simulink model "EScooter_Logical_Architecture"  (R2025b)
settings: Solver=VariableStepAuto  StartTime=0.0  StopTime=10.0  RelTol=1e-3
settings Model: Creator=louis  LastModifiedBy=louis

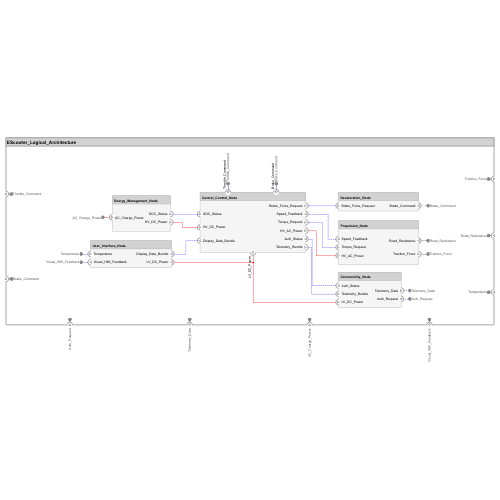
[thumbnail: Simulink's stored preview of the top-level diagram]
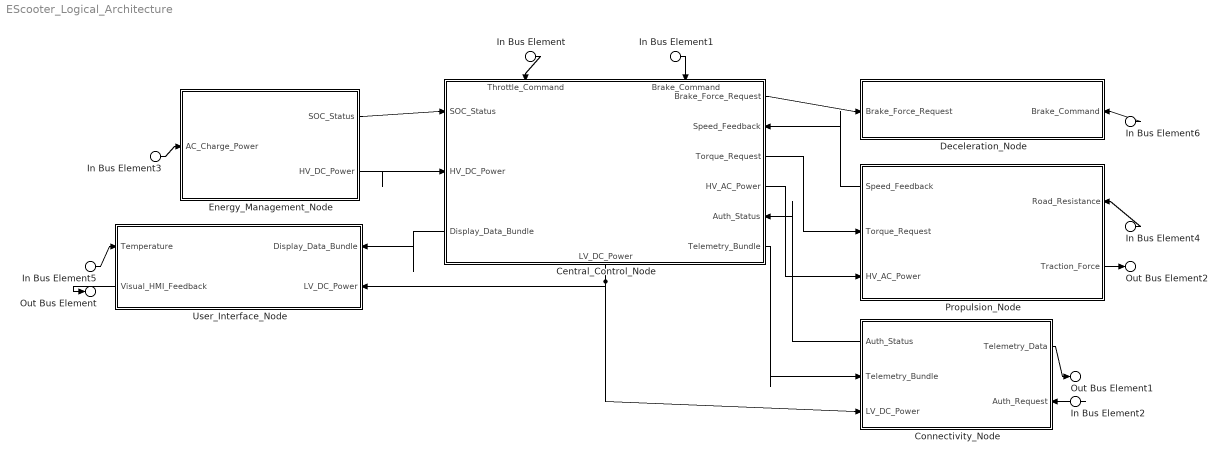
== system EScooter_Logical_Architecture ==
  In Bus Element : Inport  PortName=Throttle_Command
  In Bus Element6 : Inport  Port=2  PortName=Brake_Command
  In Bus Element1 : Inport  Port=2  PortName=Brake_Command
  In Bus Element2 : Inport  Port=3  PortName=Auth_Request
  In Bus Element3 : Inport  Port=4  PortName=AC_Charge_Power
  In Bus Element4 : Inport  Port=5  PortName=Road_Resistance
  In Bus Element5 : Inport  Port=6  PortName=Temperature
  Central_Control_Node : Subsystem
      settings: PortSchema="{\"entries\":[{\"content\":{\"headerSize\":26,\"margin\":15,\"minimumSpacing\":25,\"sides\":[{\"content\":{\"connectorIds\":[\"In6\",\"In3\",\"Out3\"]},\"type\":\"ConnectorPlacement.EquallySpacedRectSide\",\"uuid\":\"144652b9-dd85-470f-8014-e792da2fa2ac\"},{\"content\":{\"connectorIds\":[\"Out4\",\"In5\",\"Out6\",\"Out2\",\"In4\",\"Out5\"],\"side\":\"RIGHT\"},\"type\":\"ConnectorPlacement.EquallySpacedRectSide\",\"uuid\":\"d391e3f2-978f-4ccc-ab2b-52567d421a28\"},{\"content\":{\"connectorIds\":[\"In1\",\"In2\"],\"side\":\"TOP\"},\"type\":\"ConnectorPlacement.EquallySpacedRectSide\",\"uuid\":\"a45f99b3-1281-4051-bb9b-2205db18ec2a\"},{\"content\":{\"connectorIds\":[\"Out1\"],\"side\":\"BOTTOM\"},\"type\":\"ConnectorPlacement.EquallySpacedRectSide\",\"uuid\":\"be097ea3-5c6b-435f-9d5e-6a4f101ead8d\"}]},\"type\":\"ConnectorPlacement.EquallySpacedConnector\",\"uuid\":\"69c8647b-5d40-4da9-a90b-a75e053ae147\"}],\"packageUris\":[\"http://schema.mathworks.com/mf0/Connector/R2020b\"],\"version\":\"1.0\"}"
  Connectivity_Node : Subsystem
      settings: PortSchema="{\"entries\":[{\"content\":{\"headerSize\":26,\"margin\":15,\"minimumSpacing\":25,\"sides\":[{\"content\":{\"connectorIds\":[\"Out2\",\"In3\",\"In2\"]},\"type\":\"ConnectorPlacement.EquallySpacedRectSide\",\"uuid\":\"144652b9-dd85-470f-8014-e792da2fa2ac\"},{\"content\":{\"connectorIds\":[\"Out1\",\"In1\"],\"side\":\"RIGHT\"},\"type\":\"ConnectorPlacement.EquallySpacedRectSide\",\"uuid\":\"d391e3f2-978f-4ccc-ab2b-52567d421a28\"},{\"content\":{\"side\":\"TOP\"},\"type\":\"ConnectorPlacement.EquallySpacedRectSide\",\"uuid\":\"a45f99b3-1281-4051-bb9b-2205db18ec2a\"},{\"content\":{\"side\":\"BOTTOM\"},\"type\":\"ConnectorPlacement.EquallySpacedRectSide\",\"uuid\":\"4c3afbfa-e7d8-4b27-9477-116bc0ba0eb7\"}]},\"type\":\"ConnectorPlacement.EquallySpacedConnector\",\"uuid\":\"69c8647b-5d40-4da9-a90b-a75e053ae147\"}],\"packageUris\":[\"http://schema.mathworks.com/mf0/Connector/R2020b\"],\"version\":\"1.0\"}"
  Deceleration_Node : Subsystem
      settings: PortSchema="{\"entries\":[{\"content\":{\"headerSize\":26,\"margin\":15,\"minimumSpacing\":25,\"sides\":[{\"content\":{\"connectorIds\":[\"In2\"]},\"type\":\"ConnectorPlacement.EquallySpacedRectSide\",\"uuid\":\"144652b9-dd85-470f-8014-e792da2fa2ac\"},{\"content\":{\"connectorIds\":[\"In1\"],\"side\":\"RIGHT\"},\"type\":\"ConnectorPlacement.EquallySpacedRectSide\",\"uuid\":\"d391e3f2-978f-4ccc-ab2b-52567d421a28\"},{\"content\":{\"side\":\"TOP\"},\"type\":\"ConnectorPlacement.EquallySpacedRectSide\",\"uuid\":\"a45f99b3-1281-4051-bb9b-2205db18ec2a\"}]},\"type\":\"ConnectorPlacement.EquallySpacedConnector\",\"uuid\":\"69c8647b-5d40-4da9-a90b-a75e053ae147\"}],\"packageUris\":[\"http://schema.mathworks.com/mf0/Connector/R2020b\"],\"version\":\"1.0\"}"
  Energy_Management_Node : Subsystem
      settings: PortSchema="{\"entries\":[{\"content\":{\"headerSize\":26,\"margin\":15,\"minimumSpacing\":25,\"sides\":[{\"content\":{\"connectorIds\":[\"In1\"]},\"type\":\"ConnectorPlacement.EquallySpacedRectSide\",\"uuid\":\"144652b9-dd85-470f-8014-e792da2fa2ac\"},{\"content\":{\"connectorIds\":[\"Out1\",\"Out2\"],\"side\":\"RIGHT\"},\"type\":\"ConnectorPlacement.EquallySpacedRectSide\",\"uuid\":\"d391e3f2-978f-4ccc-ab2b-52567d421a28\"},{\"content\":{\"side\":\"TOP\"},\"type\":\"ConnectorPlacement.EquallySpacedRectSide\",\"uuid\":\"a45f99b3-1281-4051-bb9b-2205db18ec2a\"}]},\"type\":\"ConnectorPlacement.EquallySpacedConnector\",\"uuid\":\"69c8647b-5d40-4da9-a90b-a75e053ae147\"}],\"packageUris\":[\"http://schema.mathworks.com/mf0/Connector/R2020b\"],\"version\":\"1.0\"}"
  Propulsion_Node : Subsystem
      settings: PortSchema="{\"entries\":[{\"content\":{\"headerSize\":26,\"margin\":15,\"minimumSpacing\":25,\"sides\":[{\"content\":{\"connectorIds\":[\"Out1\",\"In1\",\"In3\"]},\"type\":\"ConnectorPlacement.EquallySpacedRectSide\",\"uuid\":\"144652b9-dd85-470f-8014-e792da2fa2ac\"},{\"content\":{\"connectorIds\":[\"In2\",\"Out2\"],\"side\":\"RIGHT\"},\"type\":\"ConnectorPlacement.EquallySpacedRectSide\",\"uuid\":\"d391e3f2-978f-4ccc-ab2b-52567d421a28\"},{\"content\":{\"side\":\"TOP\"},\"type\":\"ConnectorPlacement.EquallySpacedRectSide\",\"uuid\":\"a45f99b3-1281-4051-bb9b-2205db18ec2a\"}]},\"type\":\"ConnectorPlacement.EquallySpacedConnector\",\"uuid\":\"69c8647b-5d40-4da9-a90b-a75e053ae147\"}],\"packageUris\":[\"http://schema.mathworks.com/mf0/Connector/R2020b\"],\"version\":\"1.0\"}"
  User_Interface_Node : Subsystem
      settings: PortSchema="{\"entries\":[{\"content\":{\"headerSize\":26,\"margin\":15,\"minimumSpacing\":25,\"sides\":[{\"content\":{\"connectorIds\":[\"In1\",\"Out1\"]},\"type\":\"ConnectorPlacement.EquallySpacedRectSide\",\"uuid\":\"144652b9-dd85-470f-8014-e792da2fa2ac\"},{\"content\":{\"connectorIds\":[\"In3\",\"In2\"],\"side\":\"RIGHT\"},\"type\":\"ConnectorPlacement.EquallySpacedRectSide\",\"uuid\":\"d391e3f2-978f-4ccc-ab2b-52567d421a28\"},{\"content\":{\"side\":\"TOP\"},\"type\":\"ConnectorPlacement.EquallySpacedRectSide\",\"uuid\":\"a45f99b3-1281-4051-bb9b-2205db18ec2a\"}]},\"type\":\"ConnectorPlacement.EquallySpacedConnector\",\"uuid\":\"69c8647b-5d40-4da9-a90b-a75e053ae147\"}],\"packageUris\":[\"http://schema.mathworks.com/mf0/Connector/R2020b\"],\"version\":\"1.0\"}"
  Out Bus Element : Outport  PortName=Visual_HMI_Feedback
  Out Bus Element1 : Outport  Port=2  PortName=Telemetry_Data
  Out Bus Element2 : Outport  Port=3  PortName=Traction_Force
  wires:
  Energy_Management_Node/1(SOC_Status) -> Central_Control_Node/6(SOC_Status)
  Connectivity_Node/2(Auth_Status) -> Central_Control_Node/4(Auth_Status)
  Central_Control_Node/4(Brake_Force_Request) -> Deceleration_Node/2(Brake_Force_Request)
  Propulsion_Node/1(Speed_Feedback) -> Central_Control_Node/5(Speed_Feedback)
  Central_Control_Node/3(Display_Data_Bundle) -> User_Interface_Node/3(Display_Data_Bundle)
  Central_Control_Node/5(Telemetry_Bundle) -> Connectivity_Node/3(Telemetry_Bundle)
  Central_Control_Node/6(Torque_Request) -> Propulsion_Node/1(Torque_Request)
  User_Interface_Node/1(Visual_HMI_Feedback) -> Out Bus Element/1
  In Bus Element2/1 -> Connectivity_Node/1(Auth_Request)
  Connectivity_Node/1(Telemetry_Data) -> Out Bus Element1/1
  In Bus Element3/1 -> Energy_Management_Node/1(AC_Charge_Power)
  Propulsion_Node/2(Traction_Force) -> Out Bus Element2/1
  In Bus Element4/1 -> Propulsion_Node/2(Road_Resistance)
  In Bus Element5/1 -> User_Interface_Node/1(Temperature)
  Energy_Management_Node/2(HV_DC_Power) -> Central_Control_Node/3(HV_DC_Power)
  Central_Control_Node/2(HV_AC_Power) -> Propulsion_Node/3(HV_AC_Power)
  Central_Control_Node/1(LV_DC_Power) -> Connectivity_Node/2(LV_DC_Power), User_Interface_Node/2(LV_DC_Power)
  In Bus Element6/1 -> Deceleration_Node/1(Brake_Command)
  In Bus Element1/1 -> Central_Control_Node/2(Brake_Command)
  In Bus Element/1 -> Central_Control_Node/1(Throttle_Command)

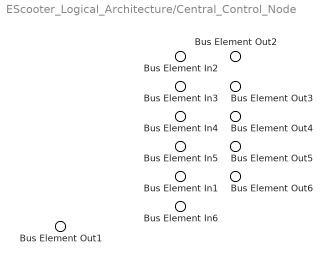
== system EScooter_Logical_Architecture/Central_Control_Node ==
  Bus Element In6 : Inport  PortName=Throttle_Command
  Bus Element In1 : Inport  Port=2  PortName=Brake_Command
  Bus Element In2 : Inport  Port=3  PortName=HV_DC_Power
  Bus Element In5 : Inport  Port=4  PortName=Auth_Status
  Bus Element In3 : Inport  Port=5  PortName=Speed_Feedback
  Bus Element In4 : Inport  Port=6  PortName=SOC_Status
  Bus Element Out6 : Outport  PortName=LV_DC_Power
  Bus Element Out5 : Outport  Port=2  PortName=HV_AC_Power
  Bus Element Out4 : Outport  Port=3  PortName=Display_Data_Bundle
  Bus Element Out2 : Outport  Port=4  PortName=Brake_Force_Request
  Bus Element Out3 : Outport  Port=5  PortName=Telemetry_Bundle
  Bus Element Out1 : Outport  Port=6  PortName=Torque_Request

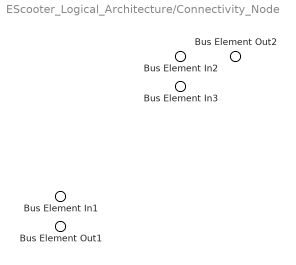
== system EScooter_Logical_Architecture/Connectivity_Node ==
  Bus Element In2 : Inport  PortName=Auth_Request
  Bus Element In3 : Inport  Port=2  PortName=LV_DC_Power
  Bus Element In1 : Inport  Port=3  PortName=Telemetry_Bundle
  Bus Element Out2 : Outport  PortName=Telemetry_Data
  Bus Element Out1 : Outport  Port=2  PortName=Auth_Status

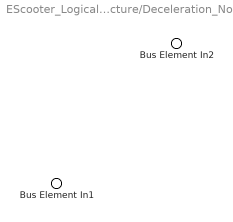
== system EScooter_Logical_Architecture/Deceleration_Node ==
  Bus Element In2 : Inport  PortName=Brake_Command
  Bus Element In1 : Inport  Port=2  PortName=Brake_Force_Request

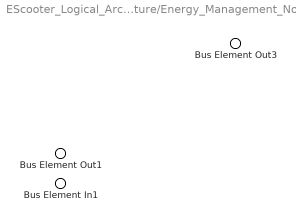
== system EScooter_Logical_Architecture/Energy_Management_Node ==
  Bus Element In1 : Inport  PortName=AC_Charge_Power
  Bus Element Out3 : Outport  PortName=SOC_Status
  Bus Element Out1 : Outport  Port=2  PortName=HV_DC_Power

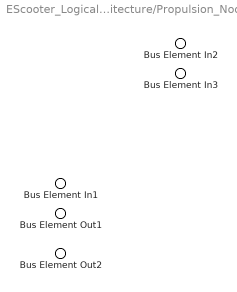
== system EScooter_Logical_Architecture/Propulsion_Node ==
  Bus Element In2 : Inport  PortName=Torque_Request
  Bus Element In3 : Inport  Port=2  PortName=Road_Resistance
  Bus Element In1 : Inport  Port=3  PortName=HV_AC_Power
  Bus Element Out1 : Outport  PortName=Speed_Feedback
  Bus Element Out2 : Outport  Port=2  PortName=Traction_Force

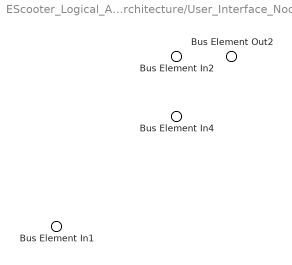
== system EScooter_Logical_Architecture/User_Interface_Node ==
  Bus Element In4 : Inport  PortName=Temperature
  Bus Element In2 : Inport  Port=2  PortName=LV_DC_Power
  Bus Element In1 : Inport  Port=3  PortName=Display_Data_Bundle
  Bus Element Out2 : Outport  PortName=Visual_HMI_Feedback
